simulink model "test"  (R2023a)
settings: Solver=FixedStepAuto  StartTime=0.0  StopTime=10.0  FixedStep=1  RelTol=1e-3
PreLoadFcn:
  | xt = importrobot('urdf\XT_PRU_noHands.urdf');
  | xt.DataFormat = 'col';
undefined symbols (not defined in the file or in its folder): SampleTime
libraries: robotmaniplib x3
settings Model: Creator=kgross  LastModifiedBy=kgross
settings SFSimCC: SimCustomInitializer="initializeMemory(\"urdf/XT_PRU_noHands.urdf\");"  SimCustomTerminator=freeMemory();  SimUserIncludeDirs=include  SimUserLibraries=build/Release/kinematics.lib  DefaultCustomCodeFunctionArrayLayout=Row-major  SimTargetLang=C++
settings SFSimCC: SimCustomHeaderCode=|
  | #include "kinematics.h"
  | #include "utils.h"

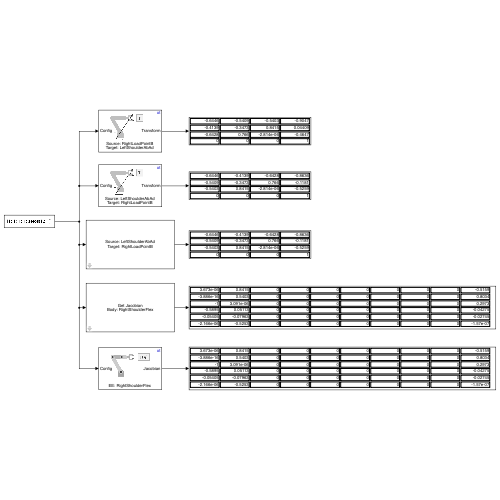
[thumbnail: Simulink's stored preview of the top-level diagram]
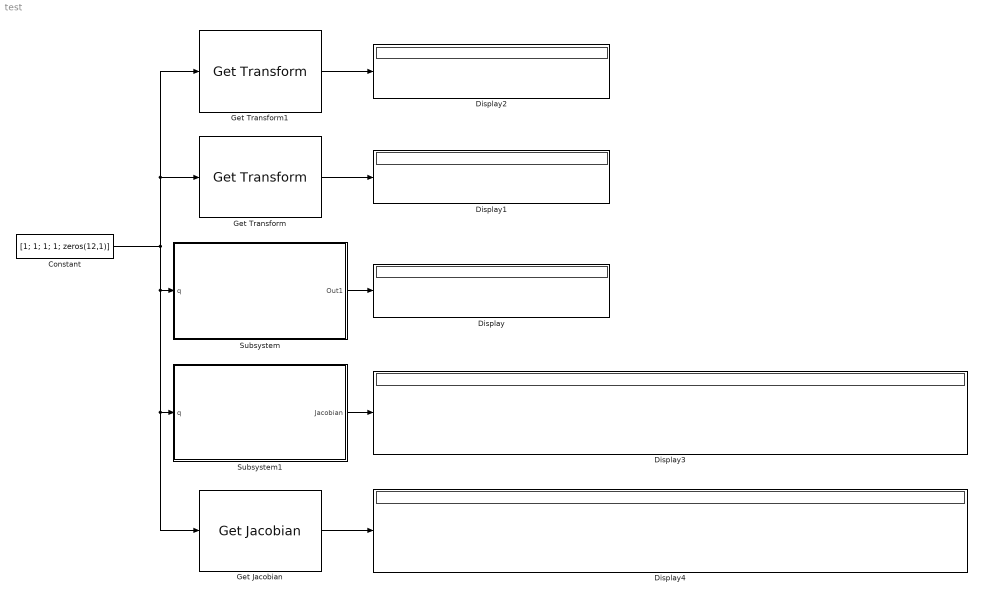
== system test ==
  Constant : Constant  Value=[1; 1; 1; 1; zeros(12,1)]
  Display{,1..4} (5 alike) : Display
  Get Jacobian : robotmaniplib/Get Jacobian  RigidBodyTree=xt  EndEffector=RightShoulderFlex  SimulateUsing=Interpreted execution
  Get Transform : robotmaniplib/Get Transform  RigidBodyTree=xt  SourceBody=LeftShoulderAbAd  TargetBody=RightLoadPointB  SimulateUsing=Interpreted execution
  Get Transform1 : robotmaniplib/Get Transform  RigidBodyTree=xt  SourceBody=RightLoadPointB  TargetBody=LeftShoulderAbAd  SimulateUsing=Interpreted execution
  Subsystem : Subsystem  mask{source='LeftShoulderAbAd', target='RightLoadPointB'}
      mask Display:
      | thisSource = get_param(gcb, "source");
      | thisTarget = get_param(gcb, "target");
      | 
      | fprintf("Source: %s\nTarget: %s", strrep(thisSource, "'", ""), strrep(thisTarget, "'", ""));
  Subsystem1 : Subsystem  mask{body='RightShoulderFlex'}
      mask Display:
      | thisSource = get_param(gcb, "body");
      | 
      | fprintf("Get Jacobian\nBody: %s", strrep(thisSource, "'", ""));
  wires:
  Constant/1 -> Get Jacobian/1, Subsystem1/1(q), Subsystem/1(q), Get Transform1/1, Get Transform/1
  Get Transform1/1 -> Display2/1
  Subsystem/1(Out1) -> Display/1
  Subsystem1/1(Jacobian) -> Display3/1
  Get Jacobian/1 -> Display4/1
  Get Transform/1 -> Display1/1

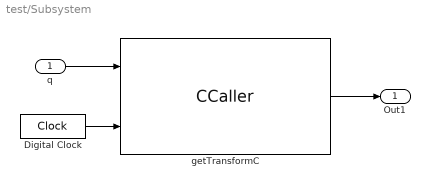
== system test/Subsystem ==
  q : Inport
  Digital Clock : DigitalClock
  getTransformC : CCaller  FunctionName=TransformFromTo  PortSpecificationStruct="%)30     .      D   8    (     @         %    \"     4    !     0         %  0 \"0    $    _    07)G3F%M90  4&]R=$YA;64 4V-O<&4     26YD97@     5'EP90      4VEZ90      27-';&]B86P   X    P    !@    @    $          4    (     0    $    !         !   0!Q    #@   #     &    \"     0         !0    @    !     0    $         $  ! '$    .    .     8    (    !          %    \"     $    %     0         0   ...(+2727 chars)"  SampleTime=SampleTime  source=uint8(source)  target=uint8(target)  SampleTime=-1
  Out1 : Outport
  wires:
  getTransformC/1 -> Out1/1
  q/1 -> getTransformC/1
  Digital Clock/1 -> getTransformC/2

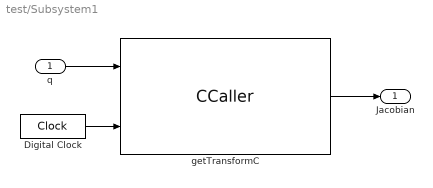
== system test/Subsystem1 ==
  q : Inport
  Digital Clock : DigitalClock
  getTransformC : CCaller  FunctionName=GetJacobianForBody  PortSpecificationStruct="%)30     .    2 <   8    (     @         %    \"     0    !     0         %  0 \"0    $    _    07)G3F%M90  4&]R=$YA;64 4V-O<&4     26YD97@     5'EP90      4VEZ90      27-';&]B86P   X    P    !@    @    $          4    (     0    $    !         !   0!Q    #@   #     &    \"     0         !0    @    !     0    $         $  ! '$    .    .     8    (    !          %    \"     $    %     0         0   ...(+2129 chars)"  SampleTime=SampleTime  bodyName=0  SampleTime=-1
  Jacobian : Outport
  wires:
  q/1 -> getTransformC/1
  getTransformC/1 -> Jacobian/1
  Digital Clock/1 -> getTransformC/2
